simulink model "adapativePIDcontrol"  (R2023b)
settings: Solver=VariableStepAuto  StartTime=0.0  StopTime=4  RelTol=1e-3
undefined symbols (not defined in the file or in its folder): J1, J2, J3, J4, J5, J6, my_gravity_torque, my_mass_matrix, my_velocity_product
settings Model: Creator=孙伟杰  LastModifiedBy=孙伟杰

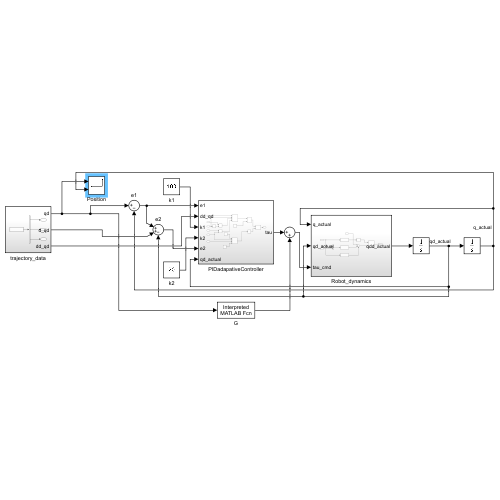
[thumbnail: Simulink's stored preview of the top-level diagram]
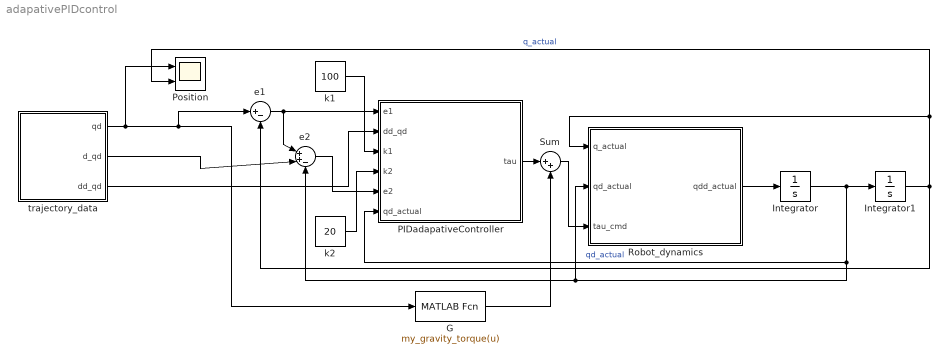
== system adapativePIDcontrol ==
  G : MATLABFcn  MATLABFcn=my_gravity_torque(u)  OutputDimensions=6
  Integrator : Integrator
  Integrator1 : Integrator
  PIDadapativeController : Subsystem
  Position : Scope  NumInputPorts=2
  Robot_dynamics : Subsystem
  Sum : Sum  Inputs=|++
  e1 : Sum  Inputs=|+-
  e2 : Sum  Inputs=|++-
  k1 : Constant  Value=100
  k2 : Constant  Value=20
  trajectory_data : Subsystem
  wires:
  trajectory_data/1(qd) -> G/1, e1/1, Position/1
  trajectory_data/2(d_qd) -> e2/2
  e1/1 -> e2/1, PIDadapativeController/1(e1)
  Integrator/1 -> PIDadapativeController/6(qd_actual), e2/3, Robot_dynamics/2(qd_actual), Integrator1/1  "qd_actual"
  Integrator1/1 -> e1/2, Position/2, Robot_dynamics/1(q_actual)  "q_actual"
  Robot_dynamics/1(qdd_actual) -> Integrator/1
  trajectory_data/3(dd_qd) -> PIDadapativeController/2(dd_qd)
  e2/1 -> PIDadapativeController/5(e2)
  k1/1 -> PIDadapativeController/3(k1)
  k2/1 -> PIDadapativeController/4(k2)
  PIDadapativeController/1(tau) -> Sum/1
  G/1 -> Sum/2
  Sum/1 -> Robot_dynamics/3(tau_cmd)

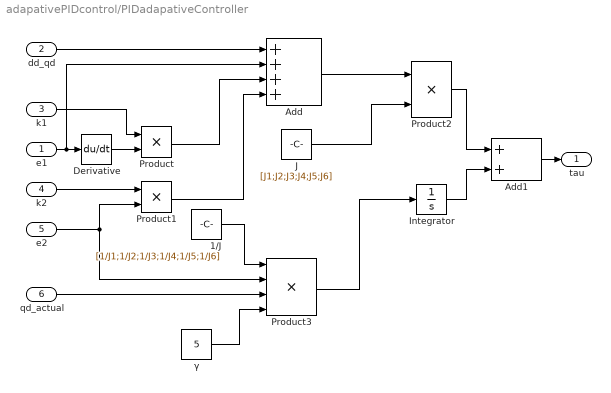
== system adapativePIDcontrol/PIDadapativeController ==
  e1 : Inport
  dd_qd : Inport  Port=2
  k1 : Inport  Port=3
  k2 : Inport  Port=4
  e2 : Inport  Port=5
  qd_actual : Inport  Port=6
  1/J : Constant  Value=[1/J1;1/J2;1/J3;1/J4;1/J5;1/J6]
  Add : Sum  Inputs=++++
  Add1 : Sum
  Derivative : Derivative
  Integrator : Integrator  LimitOutput=on  LowerSaturationLimit=0
  J : Constant  Value=[J1;J2;J3;J4;J5;J6]
  Product : Product
  Product1 : Product
  Product2 : Product
  Product3 : Product  Inputs=4
  γ : Constant  Value=5
  tau : Outport
  wires:
  dd_qd/1 -> Add/1
  e1/1 -> Add/2, Derivative/1
  k1/1 -> Product/1
  Derivative/1 -> Product/2
  Product/1 -> Add/3
  k2/1 -> Product1/1
  e2/1 -> Product1/2, Product3/2
  Product1/1 -> Add/4
  Add/1 -> Product2/1
  J/1 -> Product2/2
  qd_actual/1 -> Product3/3
  Product3/1 -> Integrator/1
  Product2/1 -> Add1/1
  Integrator/1 -> Add1/2
  Add1/1 -> tau/1
  γ/1 -> Product3/4
  1/J/1 -> Product3/1

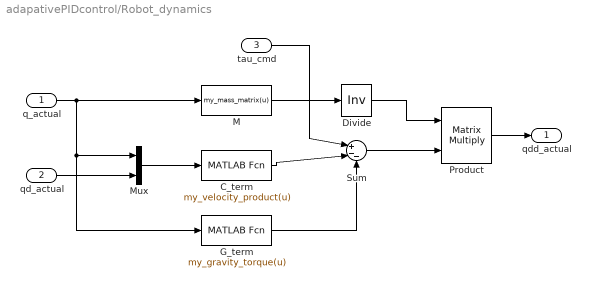
== system adapativePIDcontrol/Robot_dynamics ==
  q_actual : Inport
  qd_actual : Inport  Port=2
  tau_cmd : Inport  Port=3
  C_term : MATLABFcn  MATLABFcn=my_velocity_product(u)  OutputDimensions=6
  Divide : Product  Inputs=/  Multiplication=Matrix(*)
  G_term : MATLABFcn  MATLABFcn=my_gravity_torque(u)  OutputDimensions=6
  M : MATLABFcn  MATLABFcn=my_mass_matrix(u)  OutputDimensions=[6 6]  Output1D=off
  Mux : Mux  Inputs=2
  Product : Product  Multiplication=Matrix(*)
  Sum : Sum  Inputs=|+--
  qdd_actual : Outport
  wires:
  q_actual/1 -> G_term/1, Mux/1, M/1
  Mux/1 -> C_term/1
  qd_actual/1 -> Mux/2
  tau_cmd/1 -> Sum/1
  C_term/1 -> Sum/2
  G_term/1 -> Sum/3
  M/1 -> Divide/1
  Sum/1 -> Product/2
  Divide/1 -> Product/1
  Product/1 -> qdd_actual/1

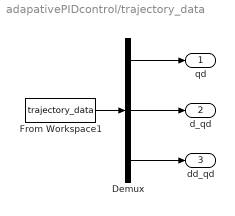
== system adapativePIDcontrol/trajectory_data ==
  Demux : Demux  Outputs=3
  From Workspace1 : FromWorkspace  VariableName=trajectory_data
  qd : Outport
  d_qd : Outport  Port=2
  dd_qd : Outport  Port=3
  wires:
  From Workspace1/1 -> Demux/1
  Demux/1 -> qd/1
  Demux/2 -> d_qd/1
  Demux/3 -> dd_qd/1
